simulink model "motorModel"  (R2017a)
settings: Solver=VariableStepAuto  StartTime=0.0  StopTime=3  MaxStep=.001  RelTol=1e-3
libraries: simulink x1
settings Model: Creator=tdarrah  LastModifiedBy=tdarrah
settings SolverCC: InitialStep=.001  ShapePreserveControl=EnableAll

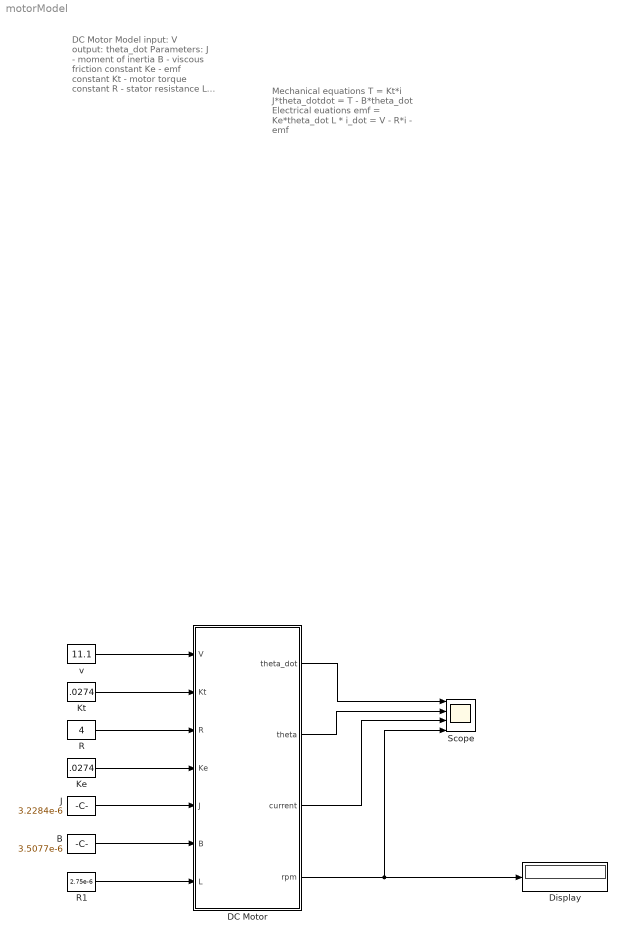
== system motorModel ==
  note: Mechanical equations
      |
      | T = Kt*i
      |
      | J*theta_dotdot = T - B*theta_dot
      |
      |
      | Electrical euations
      |
      | emf = Ke*theta_dot
      |
      | L * i_dot = V - R*i  - emf
  note: DC Motor Model
      |
      | input:
      | V
      |
      | output:
      | theta_dot
      |
      | Parameters:
      | J    - moment of inertia
      | B   - viscous friction constant
      | Ke - emf constant
      | Kt  - motor torque constant
      | R   - stator resistance
      | L   - inductance
  B : Constant  Value=3.5077e-6
  DC Motor : Subsystem
  Display : Display
  J : Constant  Value=3.2284e-6
  Ke : Constant  Value=.0274
  Kt : Constant  Value=.0274
  R : Constant  Value=4
  R1 : Constant  Value=2.75e-6
  Scope : Scope  NumInputPorts=4
  v : Constant  Value=11.1
  wires:
  DC Motor/1(theta_dot) -> Scope/1
  DC Motor/2(theta) -> Scope/2
  v/1 -> DC Motor/1(V)
  Kt/1 -> DC Motor/2(Kt)
  R/1 -> DC Motor/3(R)
  Ke/1 -> DC Motor/4(Ke)
  J/1 -> DC Motor/5(J)
  B/1 -> DC Motor/6(B)
  R1/1 -> DC Motor/7(L)
  DC Motor/4(rpm) -> Scope/4, Display/1
  DC Motor/3(current) -> Scope/3

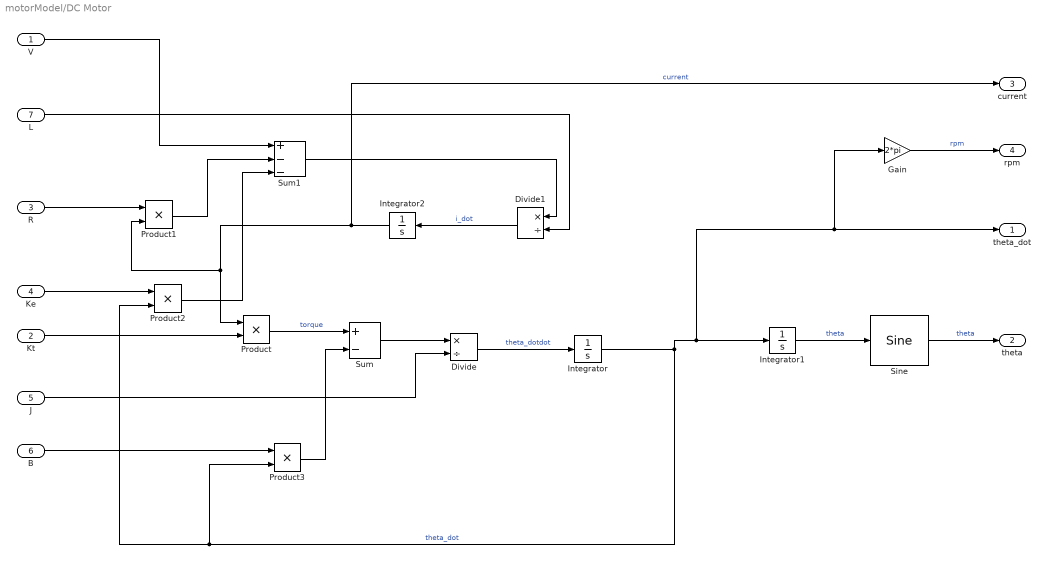
== system motorModel/DC Motor ==
  V : Inport
  Kt : Inport  Port=2
  R : Inport  Port=3
  Ke : Inport  Port=4
  J : Inport  Port=5
  B : Inport  Port=6
  L : Inport  Port=7
  Divide : Product  Inputs=*/
  Divide1 : Product  Inputs=*/
  Gain : Gain  Gain=2*pi
  Integrator : Integrator
  Integrator1 : Integrator
  Integrator2 : Integrator
  Product{,1..3} (4 alike) : Product
  Sine : simulink/Lookup Tables/Sine  Formula=sin(2*pi*u)  NumDataPoints=180  OutputWordLength=16  InternalRulePriority=Speed
      settings: SourceProductName=Simulink
  Sum : Sum  Inputs=+-
  Sum1 : Sum  Inputs=+--
  theta_dot : Outport
  theta : Outport  Port=2
  current : Outport  Port=3
  rpm : Outport  Port=4
  wires:
  Sum1/1 -> Divide1/1
  Kt/1 -> Product/2
  Product/1 -> Sum/1  "torque"
  Product1/1 -> Sum1/2
  V/1 -> Sum1/1
  Divide/1 -> Integrator/1  "theta_dotdot"
  Integrator/1 -> Gain/1, theta_dot/1, Integrator1/1, Product3/2, Product2/2  "theta_dot"
  Integrator2/1 -> current/1, Product1/2, Product/1  "current"
  Integrator1/1 -> Sine/1  "theta"
  Divide1/1 -> Integrator2/1  "i_dot"
  Sum/1 -> Divide/1
  R/1 -> Product1/1
  Sine/1 -> theta/1  "theta"
  Ke/1 -> Product2/1
  Product2/1 -> Sum1/3
  J/1 -> Divide/2
  B/1 -> Product3/1
  Product3/1 -> Sum/2
  L/1 -> Divide1/2
  Gain/1 -> rpm/1  "rpm"
